simulink model "EVX_Lap_Simulation 2"  (R2018b)
settings: Solver=FixedStepAuto  StartTime=0  StopTime=120  FixedStep=0.001  MaxStep=0.01  RelTol=1e-2
values from neighbouring files (symbols this model uses):
  velocity_dnew = velocity_d + 0.4 .* (velocity_dmax - velocity_d)    [Run_Sim(with_fmincon).m]
undefined symbols (not defined in the file or in its folder): dist, theta_d
libraries: simulink x1
(part 2 of 3)

== system EVX_Lap_Simulation 2/EVX_Vehicle_Model/Subsystem1 ==
  Tyre Coefficients : Inport
  Tyre Dynamics : Inport  Port=2
  Bus Creator : BusCreator  Inputs=3
  Bus Selector : BusSelector  OutputSignals=Fzo,Ro,q_Bz1,q_Bz2,q_Bz3,q_Bz4,q_Bz5,q_Bz9,q_Bz10,q_Cz1,q_Dz1,q_Dz2,q_Dz3,q_Dz4,q_Dz6,q_Dz7,q_Dz8,q_Dz9,q_Ez1,q_Ez2,q_Ez3,q_Ez4,q_Ez5,q_Hz1,q_Hz2,q_Hz3,q_Hz4,p_Cy1,p_Dy1,p_Dy2,p_Dy3,p_Ey1,p_Ey2,p_Ey3,p_Ey4,p_Ky1,p_Ky2,p_Ky3,p_Hy1,p_Hy2,p_Hy3,p_Vy1,p_Vy2,p_Vy3,p_Vy4,p_Cx1,p_Dx1,p_Dx2,p_Ex1,p_Ex2,p_Ex3,p_Ex4,p_Kx1,p_Kx2,p_Kx3,p_Hx1,p_Hx2,p_Vx1,p_Vx2
  Bus Selector1 : BusSelector  OutputSignals=x_WFR,xdot_WFR,signal3.k_TFR,signal3.c_TFR,signal3.gamma_FR,signal4.ratio_FR,signal4.angle_FR,mu_scaling
  Constant : Constant  Value=0
  MATLAB Function : MATLAB Function  TreatAsAtomicUnit=on
  MATLAB Function8 : MATLAB Function  TreatAsAtomicUnit=on
  Memory1 : Memory
  Multiply : Product  Inputs=3
  Multiply1 : Product  Inputs=3
  Scope : Scope
  Scope1 : Scope  NumInputPorts=3
  Output Forces : Outport
  wires:
  Bus Creator/1 -> Scope/1, Output Forces/1
  Tyre Coefficients/1 -> Bus Selector/1
  Bus Selector/1 -> MATLAB Function8/5(Fzo)  "<Fzo>"
  Bus Selector/2 -> MATLAB Function8/6(Ro)  "<Ro>"
  Tyre Dynamics/1 -> Memory1/1
  Bus Selector1/1 -> MATLAB Function/1(x)  "<x_WFR>"
  Bus Selector1/2 -> MATLAB Function/2(xdot)  "<xdot_WFR>"
  MATLAB Function/1(F_z) -> Multiply1/2, Multiply/2, Scope1/1, MATLAB Function8/1(Fz)
  Bus Selector1/3 -> MATLAB Function/3(k)  "<k_TFR>"
  Bus Selector1/4 -> MATLAB Function/4(c)  "<c_TFR>"
  Bus Selector1/5 -> MATLAB Function8/4(gam)  "<gamma_FR>"
  Bus Selector/3 -> MATLAB Function8/7(q_Bz1)  "<q_Bz1>"
  Bus Selector/4 -> MATLAB Function8/8(q_Bz2)  "<q_Bz2>"
  Bus Selector/5 -> MATLAB Function8/9(q_Bz3)  "<q_Bz3>"
  Bus Selector/6 -> MATLAB Function8/10(q_Bz4)  "<q_Bz4>"
  Bus Selector/7 -> MATLAB Function8/11(q_Bz5)  "<q_Bz5>"
  Bus Selector/8 -> MATLAB Function8/12(q_Bz9)  "<q_Bz9>"
  Bus Selector/9 -> MATLAB Function8/13(q_Bz10)  "<q_Bz10>"
  Bus Selector/10 -> MATLAB Function8/14(q_Cz1)  "<q_Cz1>"
  Bus Selector/11 -> MATLAB Function8/15(q_Dz1)  "<q_Dz1>"
  Bus Selector/12 -> MATLAB Function8/16(q_Dz2)  "<q_Dz2>"
  Bus Selector/13 -> MATLAB Function8/17(q_Dz3)  "<q_Dz3>"
  Bus Selector/14 -> MATLAB Function8/18(q_Dz4)  "<q_Dz4>"
  Bus Selector/15 -> MATLAB Function8/19(q_Dz6)  "<q_Dz6>"
  Bus Selector/16 -> MATLAB Function8/20(q_Dz7)  "<q_Dz7>"
  Bus Selector/17 -> MATLAB Function8/21(q_Dz8)  "<q_Dz8>"
  Bus Selector/18 -> MATLAB Function8/22(q_Dz9)  "<q_Dz9>"
  Bus Selector/19 -> MATLAB Function8/23(q_Ez1)  "<q_Ez1>"
  Bus Selector/20 -> MATLAB Function8/24(q_Ez2)  "<q_Ez2>"
  Bus Selector/21 -> MATLAB Function8/25(q_Ez3)  "<q_Ez3>"
  Bus Selector/22 -> MATLAB Function8/26(q_Ez4)  "<q_Ez4>"
  Bus Selector/23 -> MATLAB Function8/27(q_Ez5)  "<q_Ez5>"
  Bus Selector/24 -> MATLAB Function8/28(q_Hz1)  "<q_Hz1>"
  Bus Selector/25 -> MATLAB Function8/29(q_Hz2)  "<q_Hz2>"
  Bus Selector/26 -> MATLAB Function8/30(q_Hz3)  "<q_Hz3>"
  Bus Selector/27 -> MATLAB Function8/31(q_Hz4)  "<q_Hz4>"
  Bus Selector/28 -> MATLAB Function8/32(p_Cy1)  "<p_Cy1>"
  Bus Selector/29 -> MATLAB Function8/33(p_Dy1)  "<p_Dy1>"
  Bus Selector/30 -> MATLAB Function8/34(p_Dy2)  "<p_Dy2>"
  Bus Selector/31 -> MATLAB Function8/35(p_Dy3)  "<p_Dy3>"
  Bus Selector/32 -> MATLAB Function8/36(p_Ey1)  "<p_Ey1>"
  Bus Selector/33 -> MATLAB Function8/37(p_Ey2)  "<p_Ey2>"
  Bus Selector/34 -> MATLAB Function8/38(p_Ey3)  "<p_Ey3>"
  Bus Selector/35 -> MATLAB Function8/39(p_Ey4)  "<p_Ey4>"
  Bus Selector/36 -> MATLAB Function8/40(p_Ky1)  "<p_Ky1>"
  Bus Selector/37 -> MATLAB Function8/41(p_Ky2)  "<p_Ky2>"
  Bus Selector/38 -> MATLAB Function8/42(p_Ky3)  "<p_Ky3>"
  Bus Selector/39 -> MATLAB Function8/43(p_Hy1)  "<p_Hy1>"
  Bus Selector/40 -> MATLAB Function8/44(p_Hy2)  "<p_Hy2>"
  Bus Selector/41 -> MATLAB Function8/45(p_Hy3)  "<p_Hy3>"
  Bus Selector/42 -> MATLAB Function8/46(p_Vy1)  "<p_Vy1>"
  Bus Selector/43 -> MATLAB Function8/47(p_Vy2)  "<p_Vy2>"
  Bus Selector/44 -> MATLAB Function8/48(p_Vy3)  "<p_Vy3>"
  Bus Selector/45 -> MATLAB Function8/49(p_Vy4)  "<p_Vy4>"
  Bus Selector/46 -> MATLAB Function8/50(p_Cx1)  "<p_Cx1>"
  Bus Selector/47 -> MATLAB Function8/51(p_Dx1)  "<p_Dx1>"
  Bus Selector/48 -> MATLAB Function8/52(p_Dx2)  "<p_Dx2>"
  Bus Selector/49 -> MATLAB Function8/53(p_Ex1)  "<p_Ex1>"
  Bus Selector/50 -> MATLAB Function8/54(p_Ex2)  "<p_Ex2>"
  Bus Selector/51 -> MATLAB Function8/55(p_Ex3)  "<p_Ex3>"
  Bus Selector/52 -> MATLAB Function8/56(p_Ex4)  "<p_Ex4>"
  Bus Selector/53 -> MATLAB Function8/57(p_Kx1)  "<p_Kx1>"
  Bus Selector/54 -> MATLAB Function8/58(p_Kx2)  "<p_Kx2>"
  Bus Selector/55 -> MATLAB Function8/59(p_Kx3)  "<p_Kx3>"
  Bus Selector/56 -> MATLAB Function8/60(p_Hx1)  "<p_Hx1>"
  Bus Selector/57 -> MATLAB Function8/61(p_Hx2)  "<p_Hx2>"
  Bus Selector/58 -> MATLAB Function8/62(p_Vx1)  "<p_Vx1>"
  Bus Selector/59 -> MATLAB Function8/63(p_Vx2)  "<p_Vx2>"
  Bus Selector1/8 -> Multiply1/1, Multiply/1, MATLAB Function8/64(car_mu_scaling)  "<mu_scaling>"
  Bus Selector1/6 -> Multiply/3, Scope1/2, MATLAB Function8/2(kappa)  "<ratio_FR>"
  Bus Selector1/7 -> Scope1/3, MATLAB Function8/3(alpha), Multiply1/3  "<angle_FR>"
  Memory1/1 -> Bus Selector1/1
  Multiply/1 -> Bus Creator/1  "Fxo"
  Multiply1/1 -> Bus Creator/2  "Fyo"
  Constant/1 -> Bus Creator/3  "Mzo"

== system EVX_Lap_Simulation 2/EVX_Vehicle_Model/Subsystem3 ==
  Steering Angle : Inport
  Bus Creator : BusCreator  Inputs=4
  Constant : Constant  Value=2
  Constant1 : Constant  Value=6
  Front/Rear Split : MATLAB Function  TreatAsAtomicUnit=on
  MATLAB Function : MATLAB Function  TreatAsAtomicUnit=on
  MATLAB Function1 : MATLAB Function  TreatAsAtomicUnit=on
  Wheel Angles : Outport
  wires:
  Steering Angle/1 -> Front/Rear Split/1(Angle)
  Front/Rear Split/1(Steering_F) -> MATLAB Function/1(Steering_F)
  Front/Rear Split/2(Steering_R) -> MATLAB Function1/1(Steering_R)
  Constant/1 -> MATLAB Function/2(Ratio)
  Constant1/1 -> MATLAB Function1/2(Ratio)
  MATLAB Function/1(S_FR) -> Bus Creator/1
  MATLAB Function1/1(S_RR) -> Bus Creator/3
  MATLAB Function1/2(S_RL) -> Bus Creator/4
  Bus Creator/1 -> Wheel Angles/1
  MATLAB Function/2(S_FL) -> Bus Creator/2

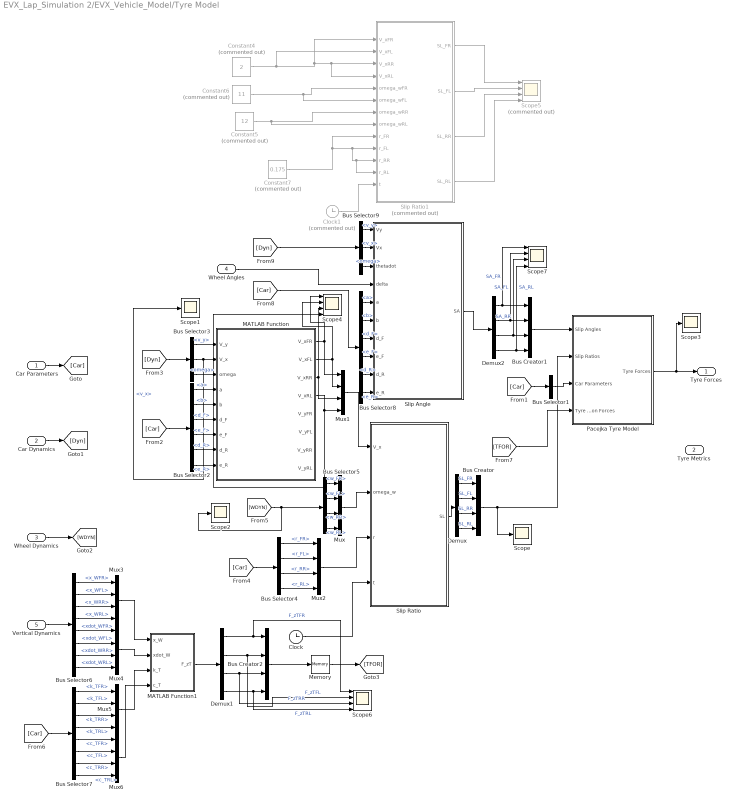
== system EVX_Lap_Simulation 2/EVX_Vehicle_Model/Tyre Model ==
  Car Parameters : Inport
  Car Dynamics : Inport  Port=2
  Wheel Dynamics : Inport  Port=3
  Wheel Angles : Inport  Port=4
  Vertical Dynamics : Inport  Port=5
  Bus Creator : BusCreator  Inputs=4
  Bus Creator1 : BusCreator  Inputs=4
  Bus Creator2 : BusCreator  Inputs=4
  Bus Selector1 : BusSelector  OutputSignals=Chassis Param,Suspension Param  OutputAsBus=on
  Bus Selector2 : BusSelector  OutputSignals=Chassis Param.a,Chassis Param.b,Chassis Param.d_F,Chassis Param.e_F,Chassis Param.d_R,Chassis Param.e_R
  Bus Selector3 : BusSelector  OutputSignals=Car Velocities.v_y,Car Velocities.v_x,Car Velocities.omega
  Bus Selector4 : BusSelector  OutputSignals=Wheel Param.r_FR,Wheel Param.r_FL,Wheel Param.r_RR,Wheel Param.r_RL
  Bus Selector5 : BusSelector  OutputSignals=w.w_FR,w.w_FL,w.w_RR,w.w_RL
  Bus Selector6 : BusSelector  OutputSignals=V_Disp.x_WFR,V_Disp.x_WFL,V_Disp.x_WRR,V_Disp.x_WRL,V_Vel.xdot_WFR,V_Vel.xdot_WFL,V_Vel.xdot_WRR,V_Vel.xdot_WRL
  Bus Selector7 : BusSelector  OutputSignals=Suspension Param.k_TFR,Suspension Param.k_TFL,Suspension Param.k_TRR,Suspension Param.k_TRL,Suspension Param.c_TFR,Suspension Param.c_TFL,Suspension Param.c_TRR,Suspension Param.c_TRL
  Bus Selector8 : BusSelector  OutputSignals=Chassis Param.a,Chassis Param.b,Chassis Param.d_F,Chassis Param.e_F,Chassis Param.d_R,Chassis Param.e_R
  Bus Selector9 : BusSelector  OutputSignals=Car Velocities.v_y,Car Velocities.v_x,Car Velocities.omega
  Clock : Clock
  Clock1 : Clock  Commented=on
  Constant4 : Constant  Commented=on  Value=2
  Constant5 : Constant  Commented=on  Value=12
  Constant6 : Constant  Commented=on  Value=11
  Constant7 : Constant  Commented=on  Value=0.175
  Demux : Demux
  Demux1 : Demux
  Demux2 : Demux
  MATLAB Function : MATLAB Function  TreatAsAtomicUnit=on
  MATLAB Function1 : MATLAB Function  TreatAsAtomicUnit=on
  Memory : Memory
  Mux{,1..6} (7 alike) : Mux
  Pacejka Tyre Model : Subsystem
  Scope{,1..3} (4 alike) : Scope
  Scope4 : Scope  NumInputPorts=4
  Scope5 : Scope  Commented=on  NumInputPorts=4
  Scope6 : Scope  NumInputPorts=4
  Scope7 : Scope  NumInputPorts=4
  Slip Angle : MATLAB Function  TreatAsAtomicUnit=on
  Slip Ratio : MATLAB Function  TreatAsAtomicUnit=on
  Slip Ratio1 : MATLAB Function  Commented=on  TreatAsAtomicUnit=on
  Tyre Forces : Outport
  Tyre Metrics : Outport  Port=2
  wires:
  Car Parameters/1 -> [Car]
  [Car] -> Bus Selector1/1
  [Car] -> Bus Selector2/1
  Bus Selector2/1 -> MATLAB Function/4(a)  "<a>"
  Bus Selector2/2 -> MATLAB Function/5(b)  "<b>"
  Bus Selector2/3 -> MATLAB Function/6(d_F)  "<d_F>"
  Bus Selector2/4 -> MATLAB Function/7(e_F)  "<e_F>"
  Bus Selector2/5 -> MATLAB Function/8(d_R)  "<d_R>"
  Bus Selector2/6 -> MATLAB Function/9(e_R)  "<e_R>"
  Car Dynamics/1 -> [Dyn]
  [Dyn] -> Bus Selector3/1
  Bus Selector3/3 -> MATLAB Function/3(omega)  "<omega>"
  Bus Selector3/1 -> MATLAB Function/1(V_y)  "<v_y>"
  Bus Selector3/2 -> Scope1/1, MATLAB Function/2(V_x)  "<v_x>"
  MATLAB Function/1(V_xFR) -> Scope4/1, Mux1/1
  MATLAB Function/2(V_xFL) -> Scope4/2, Mux1/2
  MATLAB Function/3(V_xRR) -> Scope4/3, Mux1/3
  MATLAB Function/4(V_xRL) -> Mux1/4, Scope4/4
  [Car] -> Bus Selector4/1
  Wheel Dynamics/1 -> [WDYN]
  [WDYN] -> Scope2/1, Bus Selector5/1
  Pacejka Tyre Model/1(Tyre Forces) -> Scope3/1, Tyre Forces/1
  Bus Selector1/1 -> Pacejka Tyre Model/3(Car Parameters)
  Bus Creator/1 -> Scope/1, Pacejka Tyre Model/2(Slip Ratios)
  Bus Creator1/1 -> Pacejka Tyre Model/1(Slip Angles)
  [TFOR] -> Pacejka Tyre Model/4(Tyre Reaction Forces)
  Clock/1 -> Slip Ratio/4(t)
  Constant4/1 -> Slip Ratio1/2(V_xFL), Slip Ratio1/1(V_xFR), Slip Ratio1/4(V_xRL), Slip Ratio1/3(V_xRR)
  Constant5/1 -> Slip Ratio1/8(omega_wRL), Slip Ratio1/7(omega_wRR)
  Constant6/1 -> Slip Ratio1/6(omega_wFL), Slip Ratio1/5(omega_wFR)
  Constant7/1 -> Slip Ratio1/12(r_RL), Slip Ratio1/11(r_RR), Slip Ratio1/10(r_FL), Slip Ratio1/9(r_FR)
  Clock1/1 -> Slip Ratio1/13(t)
  Slip Ratio1/1(SL_FR) -> Scope5/1
  Slip Ratio1/2(SL_FL) -> Scope5/2
  Slip Ratio1/3(SL_RR) -> Scope5/3
  Slip Ratio1/4(SL_RL) -> Scope5/4
  Bus Selector5/4 -> Mux/4  "<w_RL>"
  Bus Selector5/1 -> Mux/1  "<w_FR>"
  Bus Selector5/2 -> Mux/2  "<w_FL>"
  Bus Selector5/3 -> Mux/3  "<w_RR>"
  Mux/1 -> Slip Ratio/2(omega_w)
  Mux1/1 -> Slip Ratio/1(V_x)
  Bus Selector4/1 -> Mux2/1  "<r_FR>"
  Bus Selector4/2 -> Mux2/2  "<r_FL>"
  Bus Selector4/3 -> Mux2/3  "<r_RR>"
  Bus Selector4/4 -> Mux2/4  "<r_RL>"
  Mux2/1 -> Slip Ratio/3(r)
  Slip Ratio/1(SL) -> Demux/1
  Demux/1 -> Bus Creator/1  "SL_FR"
  Demux/2 -> Bus Creator/2  "SL_FL"
  Demux/3 -> Bus Creator/3  "SL_RR"
  Demux/4 -> Bus Creator/4  "SL_RL"
  Vertical Dynamics/1 -> Bus Selector6/1
  Bus Selector6/1 -> Mux3/1  "<x_WFR>"
  Bus Selector6/2 -> Mux3/2  "<x_WFL>"
  Bus Selector6/3 -> Mux3/3  "<x_WRR>"
  Bus Selector6/4 -> Mux3/4  "<x_WRL>"
  Bus Selector6/5 -> Mux4/1  "<xdot_WFR>"
  Bus Selector6/6 -> Mux4/2  "<xdot_WFL>"
  Bus Selector6/7 -> Mux4/3  "<xdot_WRR>"
  Bus Selector6/8 -> Mux4/4  "<xdot_WRL>"
  [Car] -> Bus Selector7/1
  Bus Selector7/1 -> Mux5/1  "<k_TFR>"
  Bus Selector7/2 -> Mux5/2  "<k_TFL>"
  Bus Selector7/3 -> Mux5/3  "<k_TRR>"
  Bus Selector7/4 -> Mux5/4  "<k_TRL>"
  Bus Selector7/5 -> Mux6/1  "<c_TFR>"
  Bus Selector7/6 -> Mux6/2  "<c_TFL>"
  Bus Selector7/7 -> Mux6/3  "<c_TRR>"
  Bus Selector7/8 -> Mux6/4  "<c_TRL>"
  Mux3/1 -> MATLAB Function1/1(x_W)
  Mux4/1 -> MATLAB Function1/2(xdot_W)
  Mux5/1 -> MATLAB Function1/3(k_T)
  Mux6/1 -> MATLAB Function1/4(c_T)
  MATLAB Function1/1(F_zT) -> Demux1/1
  Demux1/1 -> Scope6/1, Bus Creator2/1  "F_zTFR"
  Demux1/2 -> Scope6/2, Bus Creator2/2  "F_zTFL"
  Demux1/3 -> Scope6/3, Bus Creator2/3  "F_zTRR"
  Demux1/4 -> Scope6/4, Bus Creator2/4  "F_zTRL"
  Bus Creator2/1 -> Memory/1
  Memory/1 -> [TFOR]
  [Car] -> Bus Selector8/1
  Bus Selector8/1 -> Slip Angle/5(a)  "<a>"
  Bus Selector8/2 -> Slip Angle/6(b)  "<b>"
  Bus Selector8/3 -> Slip Angle/7(d_F)  "<d_F>"
  Bus Selector8/4 -> Slip Angle/8(e_F)  "<e_F>"
  Bus Selector8/5 -> Slip Angle/9(d_R)  "<d_R>"
  Bus Selector8/6 -> Slip Angle/10(e_R)  "<e_R>"
  [Dyn] -> Bus Selector9/1
  Bus Selector9/3 -> Slip Angle/3(thetadot)  "<omega>"
  Wheel Angles/1 -> Slip Angle/4(delta)
  Slip Angle/1(SA) -> Demux2/1
  Demux2/1 -> Scope7/1, Bus Creator1/1  "SA_FR"
  Demux2/2 -> Scope7/2, Bus Creator1/2  "SA_FL"
  Demux2/3 -> Scope7/3, Bus Creator1/3  "SA_RR"
  Demux2/4 -> Scope7/4, Bus Creator1/4  "SA_RL"
  Bus Selector9/2 -> Slip Angle/2(Vx)  "<v_x>"
  Bus Selector9/1 -> Slip Angle/1(Vy)  "<v_y>"

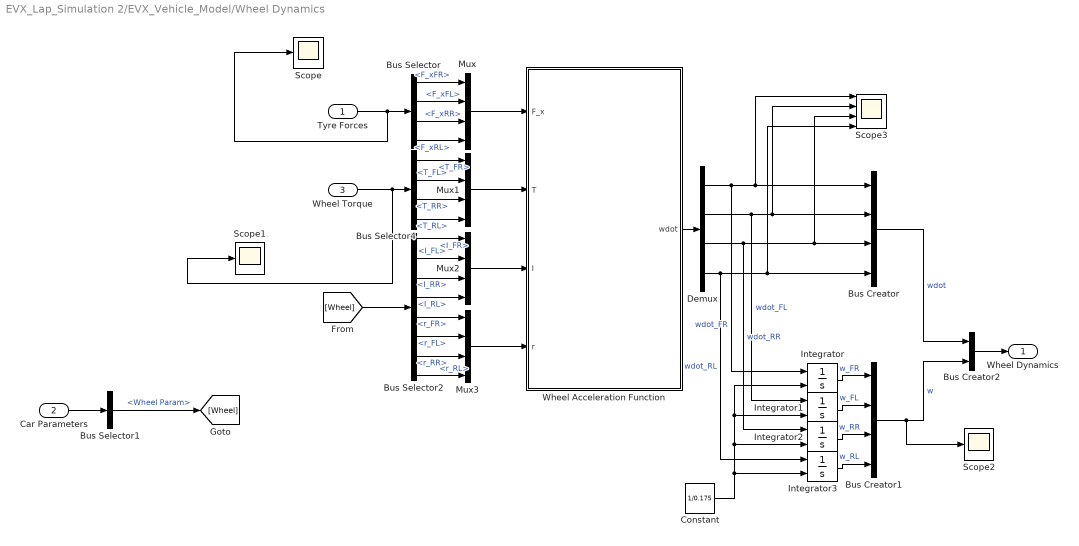
== system EVX_Lap_Simulation 2/EVX_Vehicle_Model/Wheel Dynamics ==
  Tyre Forces : Inport
  Car Parameters : Inport  Port=2
  Wheel Torque : Inport  Port=3
  Bus Creator : BusCreator  Inputs=4
  Bus Creator1 : BusCreator  Inputs=4
  Bus Creator2 : BusCreator  Inputs=2
  Bus Selector : BusSelector  OutputSignals=F_x.F_xFR,F_x.F_xFL,F_x.F_xRR,F_x.F_xRL
  Bus Selector1 : BusSelector  OutputSignals=Wheel Param
  Bus Selector2 : BusSelector  OutputSignals=I_FR,I_FL,I_RR,I_RL,r_FR,r_FL,r_RR,r_RL
  Bus Selector4 : BusSelector  OutputSignals=T_FR,T_FL,T_RR,T_RL
  Constant : Constant  Value=1/0.175
  Demux : Demux
  Integrator{,1..3} (4 alike) : Integrator  InitialConditionSource=external
  Mux{,1..3} (4 alike) : Mux
  Scope : Scope
  Scope1 : Scope
  Scope2 : Scope
  Scope3 : Scope  NumInputPorts=4
  Wheel Acceleration Function : MATLAB Function  TreatAsAtomicUnit=on
  Wheel Dynamics : Outport
  wires:
  Tyre Forces/1 -> Scope/1, Bus Selector/1
  Car Parameters/1 -> Bus Selector1/1
  Bus Selector1/1 -> [Wheel]  "<Wheel Param>"
  [Wheel] -> Bus Selector2/1
  Wheel Torque/1 -> Scope1/1, Bus Selector4/1
  Integrator/1 -> Bus Creator1/1  "w_FR"
  Integrator1/1 -> Bus Creator1/2  "w_FL"
  Integrator2/1 -> Bus Creator1/3  "w_RR"
  Integrator3/1 -> Bus Creator1/4  "w_RL"
  Bus Creator1/1 -> Scope2/1, Bus Creator2/2  "w"
  Bus Creator/1 -> Bus Creator2/1  "wdot"
  Bus Creator2/1 -> Wheel Dynamics/1
  Constant/1 -> Integrator3/2, Integrator2/2, Integrator1/2, Integrator/2
  Bus Selector/1 -> Mux/1  "<F_xFR>"
  Bus Selector/2 -> Mux/2  "<F_xFL>"
  Bus Selector/3 -> Mux/3  "<F_xRR>"
  Bus Selector/4 -> Mux/4  "<F_xRL>"
  Mux/1 -> Wheel Acceleration Function/1(F_x)
  Bus Selector4/2 -> Mux1/2  "<T_FL>"
  Bus Selector4/3 -> Mux1/3  "<T_RR>"
  Bus Selector4/4 -> Mux1/4  "<T_RL>"
  Bus Selector4/1 -> Mux1/1  "<T_FR>"
  Mux1/1 -> Wheel Acceleration Function/2(T)
  Bus Selector2/2 -> Mux2/2  "<I_FL>"
  Bus Selector2/3 -> Mux2/3  "<I_RR>"
  Bus Selector2/4 -> Mux2/4  "<I_RL>"
  Bus Selector2/1 -> Mux2/1  "<I_FR>"
  Mux2/1 -> Wheel Acceleration Function/3(I)
  Bus Selector2/5 -> Mux3/1  "<r_FR>"
  Bus Selector2/6 -> Mux3/2  "<r_FL>"
  Bus Selector2/7 -> Mux3/3  "<r_RR>"
  Bus Selector2/8 -> Mux3/4  "<r_RL>"
  Mux3/1 -> Wheel Acceleration Function/4(r)
  Wheel Acceleration Function/1(wdot) -> Demux/1
  Demux/1 -> Integrator/1, Scope3/1, Bus Creator/1  "wdot_FR"
  Demux/2 -> Integrator1/1, Scope3/2, Bus Creator/2  "wdot_FL"
  Demux/3 -> Integrator2/1, Scope3/3, Bus Creator/3  "wdot_RR"
  Demux/4 -> Integrator3/1, Scope3/4, Bus Creator/4  "wdot_RL"

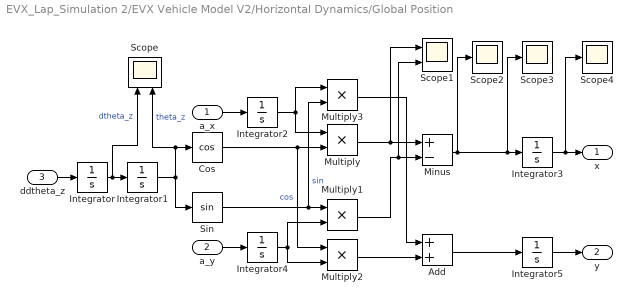
== system EVX_Lap_Simulation 2/EVX Vehicle Model V2/Horizontal Dynamics/Global Position ==
  a_x : Inport
  a_y : Inport  Port=2
  ddtheta_z : Inport  Port=3
  Add : Sum
  Cos : Trigonometry  Operator=cos
  Integrator{,1..5} (6 alike) : Integrator
  Minus : Sum  Inputs=+-
  Multiply{,1..3} (4 alike) : Product
  Scope : Scope  NumInputPorts=2
  Scope1 : Scope  NumInputPorts=2
  Scope2 : Scope
  Scope3 : Scope
  Scope4 : Scope
  Sin : Trigonometry
  x : Outport
  y : Outport  Port=2
  wires:
  ddtheta_z/1 -> Integrator/1
  Integrator/1 -> Scope/1, Integrator1/1  "dtheta_z"
  Integrator1/1 -> Scope/2, Cos/1, Sin/1  "theta_z"
  a_x/1 -> Integrator2/1
  Cos/1 -> Multiply2/1, Multiply/2  "cos"
  Sin/1 -> Multiply3/2, Multiply1/1  "sin"
  a_y/1 -> Integrator4/1
  Multiply/1 -> Scope1/1, Minus/1
  Multiply1/1 -> Scope1/2, Minus/2
  Multiply2/1 -> Add/2
  Multiply3/1 -> Add/1
  Minus/1 -> Scope3/1, Integrator3/1, Scope2/1
  Integrator3/1 -> Scope4/1, x/1
  Add/1 -> Integrator5/1
  Integrator5/1 -> y/1
  Integrator2/1 -> Multiply/1, Multiply3/1
  Integrator4/1 -> Multiply2/2, Multiply1/2

== system EVX_Lap_Simulation 2/EVX Vehicle Model V2/Horizontal Dynamics/Local Dynamics ==
  a_x : Inport
  a_y : Inport  Port=2
  ddtheta_z : Inport  Port=3
  Bus Creator{,1..3} (4 alike) : BusCreator  Inputs=3
  Integrator{,1..5} (6 alike) : Integrator
  Scope{,1..3} (4 alike) : Scope
  To Workspace : ToWorkspace  VariableName=dist_log  SaveFormat=Timeseries  SampleTime=-1
  Local Dynamics : Outport
  wires:
  Integrator/1 -> Bus Creator1/1, Scope/1, Integrator3/1  "v_x"
  Integrator2/1 -> Scope3/1, Bus Creator1/3, Integrator5/1  "dtheta_z"
  Integrator1/1 -> Bus Creator1/2, Scope2/1, Integrator4/1  "v_y"
  a_x/1 -> Bus Creator/1, Integrator/1
  a_y/1 -> Bus Creator/2, Integrator1/1
  ddtheta_z/1 -> Bus Creator/3, Integrator2/1
  Integrator4/1 -> Bus Creator2/2  "d_y"
  Integrator3/1 -> To Workspace/1, Scope1/1, Bus Creator2/1  "d_x"
  Integrator5/1 -> Bus Creator2/3  "theta_z"
  Bus Creator1/1 -> Bus Creator3/2  "Velocities"
  Bus Creator/1 -> Bus Creator3/1  "Accelerations"
  Bus Creator2/1 -> Bus Creator3/3  "Displacements"
  Bus Creator3/1 -> Local Dynamics/1

== system EVX_Lap_Simulation 2/EVX Vehicle Model V2/Tyre Model/Pacejka Tyre Model ==
  Slip Ratios : Inport
  Slip Angles : Inport  Port=2
  Tyre Reaction Forces : Inport  Port=3
  Bus Creator : BusCreator  Inputs=3
  Demux : Demux
  Demux1 : Demux
  Demux2 : Demux
  MATLAB Function4 : MATLAB Function  TreatAsAtomicUnit=on
  Scope : Scope  NumInputPorts=4
  Scope1 : Scope
  Scope2 : Scope  NumInputPorts=4
  Scope3 : Scope  NumInputPorts=4
  To Workspace : ToWorkspace  VariableName=Fz_log  SaveFormat=Timeseries  SampleTime=-1
  Tyre Forces : Outport
  wires:
  Bus Creator/1 -> Tyre Forces/1
  Slip Ratios/1 -> MATLAB Function4/2(SL)
  Slip Angles/1 -> MATLAB Function4/1(SA)
  Tyre Reaction Forces/1 -> To Workspace/1, Scope1/1, MATLAB Function4/3(Fz)
  MATLAB Function4/1(F_x) -> Demux/1, Bus Creator/1
  MATLAB Function4/2(F_y) -> Demux2/1, Bus Creator/2
  MATLAB Function4/3(M_z) -> Demux1/1, Bus Creator/3
  Demux/1 -> Scope/1  "F_xFL"
  Demux/2 -> Scope/2  "F_xFR"
  Demux/3 -> Scope/3  "F_xRL"
  Demux/4 -> Scope/4  "F_xRR"
  Demux1/1 -> Scope2/1  "M_zFL"
  Demux1/2 -> Scope2/2  "M_zFR"
  Demux1/3 -> Scope2/3  "M_zRL"
  Demux1/4 -> Scope2/4  "M_zRR"
  Demux2/1 -> Scope3/1  "F_yFL"
  Demux2/2 -> Scope3/2  "F_yFR"
  Demux2/3 -> Scope3/3  "F_yRL"
  Demux2/4 -> Scope3/4  "F_yRR"

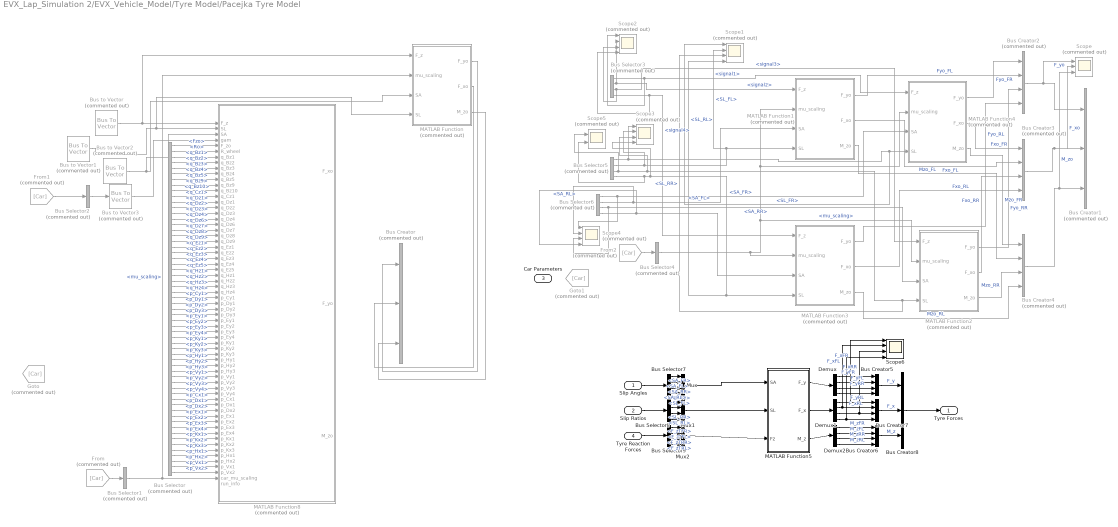
== system EVX_Lap_Simulation 2/EVX_Vehicle_Model/Tyre Model/Pacejka Tyre Model ==
  Slip Angles : Inport
  Slip Ratios : Inport  Port=2
  Car Parameters : Inport  Port=3
  Tyre Reaction Forces : Inport  Port=4
  Bus Creator : BusCreator  Commented=on  Inputs=3
  Bus Creator1 : BusCreator  Commented=on  Inputs=3
  Bus Creator2 : BusCreator  Commented=on  Inputs=4
  Bus Creator3 : BusCreator  Commented=on  Inputs=4
  Bus Creator4 : BusCreator  Commented=on  Inputs=4
  Bus Creator5 : BusCreator  Inputs=4
  Bus Creator6 : BusCreator  Inputs=4
  Bus Creator7 : BusCreator  Inputs=4
  Bus Creator8 : BusCreator  Inputs=3
  Bus Selector : BusSelector  Commented=on  OutputSignals=Fzo,Ro,q_Bz1,q_Bz2,q_Bz3,q_Bz4,q_Bz5,q_Bz9,q_Bz10,q_Cz1,q_Dz1,q_Dz2,q_Dz3,q_Dz4,q_Dz6,q_Dz7,q_Dz8,q_Dz9,q_Ez1,q_Ez2,q_Ez3,q_Ez4,q_Ez5,q_Hz1,q_Hz2,q_Hz3,q_Hz4,p_Cy1,p_Dy1,p_Dy2,p_Dy3,p_Ey1,p_Ey2,p_Ey3,p_Ey4,p_Ky1,p_Ky2,p_Ky3,p_Hy1,p_Hy2,p_Hy3,p_Vy1,p_Vy2,p_Vy3,p_Vy4,p_Cx1,p_Dx1,p_Dx2,p_Ex1,p_Ex2,p_Ex3,p_Ex4,p_Kx1,p_Kx2,p_Kx3,p_Hx1,p_Hx2,p_Vx1,p_Vx2
  Bus Selector1 : BusSelector  Commented=on  OutputSignals=Chassis Param.mu_scaling
  Bus Selector2 : BusSelector  Commented=on  OutputSignals=Suspension Param.gamma_FR,Suspension Param.gamma_FL,Suspension Param.gamma_RR,Suspension Param.gamma_RL  OutputAsBus=on
  Bus Selector3 : BusSelector  Commented=on  OutputSignals=signal1,signal2,signal3,signal4
  Bus Selector4 : BusSelector  Commented=on  OutputSignals=Chassis Param.mu_scaling
  Bus Selector5 : BusSelector  Commented=on  OutputSignals=SL_FR,SL_FL,SL_RR,SL_RL
  Bus Selector6 : BusSelector  Commented=on  OutputSignals=SA_FR,SA_FL,SA_RR,SA_RL
  Bus Selector7 : BusSelector  OutputSignals=SA_FR,SA_FL,SA_RR,SA_RL
  Bus Selector8 : BusSelector  OutputSignals=SL_FR,SL_FL,SL_RR,SL_RL
  Bus Selector9 : BusSelector  OutputSignals=F_zTFR,F_zTFL,F_zTRR,F_zTRL
  Bus to Vector{,1..3} (4 alike) : BusToVector  Commented=on
  Demux : Demux
  Demux1 : Demux
  Demux2 : Demux
  From : From  Commented=on  GotoTag=Car
  From1 : From  Commented=on  GotoTag=Car
  From2 : From  Commented=on  GotoTag=Car
  Goto : Goto  Commented=on  GotoTag=Car
  Goto1 : Goto  Commented=on  GotoTag=Car
  MATLAB Function : MATLAB Function  Commented=on  TreatAsAtomicUnit=on
  MATLAB Function1 : MATLAB Function  Commented=on  TreatAsAtomicUnit=on
  MATLAB Function2 : MATLAB Function  Commented=on  TreatAsAtomicUnit=on
  MATLAB Function3 : MATLAB Function  Commented=on  TreatAsAtomicUnit=on
  MATLAB Function4 : MATLAB Function  Commented=on  TreatAsAtomicUnit=on
  MATLAB Function5 : MATLAB Function  TreatAsAtomicUnit=on
  MATLAB Function8 : MATLAB Function  Commented=on  TreatAsAtomicUnit=on
  Mux : Mux
  Mux1 : Mux
  Mux2 : Mux
  Scope : Scope  Commented=on  NumInputPorts=3
  Scope{1..4} (4 alike) : Scope  Commented=on  NumInputPorts=4
  Scope5 : Scope  Commented=on  NumInputPorts=2
  Scope6 : Scope  NumInputPorts=4
  Tyre Forces : Outport
  wires:
  Bus Selector/1 -> MATLAB Function8/5(F_zo)  "<Fzo>"
  Bus Selector/2 -> MATLAB Function8/6(R_wheel)  "<Ro>"
  Bus Selector/3 -> MATLAB Function8/7(q_Bz1)  "<q_Bz1>"
  Bus Selector/4 -> MATLAB Function8/8(q_Bz2)  "<q_Bz2>"
  Bus Selector/5 -> MATLAB Function8/9(q_Bz3)  "<q_Bz3>"
  Bus Selector/6 -> MATLAB Function8/10(q_Bz4)  "<q_Bz4>"
  Bus Selector/7 -> MATLAB Function8/11(q_Bz5)  "<q_Bz5>"
  Bus Selector/8 -> MATLAB Function8/12(q_Bz9)  "<q_Bz9>"
  Bus Selector/9 -> MATLAB Function8/13(q_Bz10)  "<q_Bz10>"
  Bus Selector/10 -> MATLAB Function8/14(q_Cz1)  "<q_Cz1>"
  Bus Selector/11 -> MATLAB Function8/15(q_Dz1)  "<q_Dz1>"
  Bus Selector/12 -> MATLAB Function8/16(q_Dz2)  "<q_Dz2>"
  Bus Selector/13 -> MATLAB Function8/17(q_Dz3)  "<q_Dz3>"
  Bus Selector/14 -> MATLAB Function8/18(q_Dz4)  "<q_Dz4>"
  Bus Selector/15 -> MATLAB Function8/19(q_Dz6)  "<q_Dz6>"
  Bus Selector/16 -> MATLAB Function8/20(q_Dz7)  "<q_Dz7>"
  Bus Selector/17 -> MATLAB Function8/21(q_Dz8)  "<q_Dz8>"
  Bus Selector/18 -> MATLAB Function8/22(q_Dz9)  "<q_Dz9>"
  Bus Selector/19 -> MATLAB Function8/23(q_Ez1)  "<q_Ez1>"
  Bus Selector/20 -> MATLAB Function8/24(q_Ez2)  "<q_Ez2>"
  Bus Selector/21 -> MATLAB Function8/25(q_Ez3)  "<q_Ez3>"
  Bus Selector/22 -> MATLAB Function8/26(q_Ez4)  "<q_Ez4>"
  Bus Selector/23 -> MATLAB Function8/27(q_Ez5)  "<q_Ez5>"
  Bus Selector/24 -> MATLAB Function8/28(q_Hz1)  "<q_Hz1>"
  Bus Selector/25 -> MATLAB Function8/29(q_Hz2)  "<q_Hz2>"
  Bus Selector/26 -> MATLAB Function8/30(q_Hz3)  "<q_Hz3>"
  Bus Selector/27 -> MATLAB Function8/31(q_Hz4)  "<q_Hz4>"
  Bus Selector/28 -> MATLAB Function8/32(p_Cy1)  "<p_Cy1>"
  Bus Selector/29 -> MATLAB Function8/33(p_Dy1)  "<p_Dy1>"
  Bus Selector/30 -> MATLAB Function8/34(p_Dy2)  "<p_Dy2>"
  Bus Selector/31 -> MATLAB Function8/35(p_Dy3)  "<p_Dy3>"
  Bus Selector/32 -> MATLAB Function8/36(p_Ey1)  "<p_Ey1>"
  Bus Selector/33 -> MATLAB Function8/37(p_Ey2)  "<p_Ey2>"
  Bus Selector/34 -> MATLAB Function8/38(p_Ey3)  "<p_Ey3>"
  Bus Selector/35 -> MATLAB Function8/39(p_Ey4)  "<p_Ey4>"
  Bus Selector/36 -> MATLAB Function8/40(p_Ky1)  "<p_Ky1>"
  Bus Selector/37 -> MATLAB Function8/41(p_Ky2)  "<p_Ky2>"
  Bus Selector/38 -> MATLAB Function8/42(p_Ky3)  "<p_Ky3>"
  Bus Selector/39 -> MATLAB Function8/43(p_Hy1)  "<p_Hy1>"
  Bus Selector/40 -> MATLAB Function8/44(p_Hy2)  "<p_Hy2>"
  Bus Selector/41 -> MATLAB Function8/45(p_Hy3)  "<p_Hy3>"
  Bus Selector/42 -> MATLAB Function8/46(p_Vy1)  "<p_Vy1>"
  Bus Selector/43 -> MATLAB Function8/47(p_Vy2)  "<p_Vy2>"
  Bus Selector/44 -> MATLAB Function8/48(p_Vy3)  "<p_Vy3>"
  Bus Selector/45 -> MATLAB Function8/49(p_Vy4)  "<p_Vy4>"
  Bus Selector/46 -> MATLAB Function8/50(p_Cx1)  "<p_Cx1>"
  Bus Selector/47 -> MATLAB Function8/51(p_Dx1)  "<p_Dx1>"
  Bus Selector/48 -> MATLAB Function8/52(p_Dx2)  "<p_Dx2>"
  Bus Selector/49 -> MATLAB Function8/53(p_Ex1)  "<p_Ex1>"
  Bus Selector/50 -> MATLAB Function8/54(p_Ex2)  "<p_Ex2>"
  Bus Selector/51 -> MATLAB Function8/55(p_Ex3)  "<p_Ex3>"
  Bus Selector/52 -> MATLAB Function8/56(p_Ex4)  "<p_Ex4>"
  Bus Selector/53 -> MATLAB Function8/57(p_Kx1)  "<p_Kx1>"
  Bus Selector/54 -> MATLAB Function8/58(p_Kx2)  "<p_Kx2>"
  Bus Selector/55 -> MATLAB Function8/59(p_Kx3)  "<p_Kx3>"
  Bus Selector/56 -> MATLAB Function8/60(p_Hx1)  "<p_Hx1>"
  Bus Selector/57 -> MATLAB Function8/61(p_Hx2)  "<p_Hx2>"
  Bus Selector/58 -> MATLAB Function8/62(p_Vx1)  "<p_Vx1>"
  Bus Selector/59 -> MATLAB Function8/63(p_Vx2)  "<p_Vx2>"
  Bus Selector1/1 -> MATLAB Function/2(mu_scaling), MATLAB Function8/64(car_mu_scaling)  "<mu_scaling>"
  From/1 -> Bus Selector1/1
  From1/1 -> Bus Selector2/1
  Bus Selector2/1 -> Bus to Vector3/1
  Bus to Vector/1 -> MATLAB Function/1(F_z), MATLAB Function8/1(F_z)
  Bus to Vector1/1 -> MATLAB Function/4(SL), MATLAB Function8/2(SL)
  Bus to Vector2/1 -> MATLAB Function/3(SA), MATLAB Function8/3(SA)
  Bus to Vector3/1 -> MATLAB Function8/4(gam)
  MATLAB Function/1(F_yo) -> Bus Creator/1
  MATLAB Function/2(F_xo) -> Bus Creator/2
  MATLAB Function/3(M_zo) -> Bus Creator/3
  Bus Selector4/1 -> MATLAB Function3/2(mu_scaling), MATLAB Function2/2(mu_scaling), MATLAB Function1/2(mu_scaling), MATLAB Function4/2(mu_scaling)  "<mu_scaling>"
  From2/1 -> Bus Selector4/1
  Bus Selector5/1 -> Scope3/1, Scope1/1, MATLAB Function4/4(SL)  "<SL_FR>"
  Bus Selector5/2 -> Scope3/2, MATLAB Function1/4(SL), Scope1/2  "<SL_FL>"
  Bus Selector5/3 -> Scope1/3, MATLAB Function2/4(SL), Scope3/3, Scope5/1  "<SL_RR>"
  Bus Selector5/4 -> Scope5/2, Scope3/4, MATLAB Function3/4(SL), Scope1/4  "<SL_RL>"
  Bus Selector6/1 -> Scope4/1, MATLAB Function4/3(SA)  "<SA_FR>"
  Bus Selector6/2 -> Scope4/2, MATLAB Function1/3(SA)  "<SA_FL>"
  Bus Selector6/3 -> MATLAB Function2/3(SA), Scope4/3  "<SA_RR>"
  Bus Selector6/4 -> Scope4/4, MATLAB Function3/3(SA)  "<SA_RL>"
  MATLAB Function4/1(F_yo) -> Bus Creator2/1  "Fyo_FR"
  MATLAB Function1/1(F_yo) -> Bus Creator2/2  "Fyo_FL"
  MATLAB Function2/1(F_yo) -> Bus Creator2/3  "Fyo_RR"
  MATLAB Function3/1(F_yo) -> Bus Creator2/4  "Fyo_RL"
  MATLAB Function4/2(F_xo) -> Bus Creator3/1  "Fxo_FR"
  MATLAB Function1/2(F_xo) -> Bus Creator3/2  "Fxo_FL"
  MATLAB Function2/2(F_xo) -> Bus Creator3/3  "Fxo_RR"
  MATLAB Function3/2(F_xo) -> Bus Creator3/4  "Fxo_RL"
  MATLAB Function4/3(M_zo) -> Bus Creator4/1  "Mzo_FR"
  MATLAB Function1/3(M_zo) -> Bus Creator4/2  "Mzo_FL"
  MATLAB Function2/3(M_zo) -> Bus Creator4/3  "Mzo_RR"
  MATLAB Function3/3(M_zo) -> Bus Creator4/4  "Mzo_RL"
  Bus Creator3/1 -> Scope/2, Bus Creator1/2  "F_xo"
  Bus Creator2/1 -> Scope/1, Bus Creator1/1  "F_yo"
  Bus Creator4/1 -> Scope/3, Bus Creator1/3  "M_zo"
  Bus Selector3/1 -> Scope2/1, MATLAB Function4/1(F_z)  "<signal1>"
  Bus Selector3/2 -> Scope2/2, MATLAB Function1/1(F_z)  "<signal2>"
  Bus Selector3/3 -> Scope2/3, MATLAB Function2/1(F_z)  "<signal3>"
  Bus Selector3/4 -> Scope2/4, MATLAB Function3/1(F_z)  "<signal4>"
  Slip Angles/1 -> Bus Selector7/1
  Bus Selector8/2 -> Mux1/2  "<SL_FL>"
  Slip Ratios/1 -> Bus Selector8/1
  Bus Selector8/1 -> Mux1/1  "<SL_FR>"
  Bus Selector8/3 -> Mux1/3  "<SL_RR>"
  Bus Selector8/4 -> Mux1/4  "<SL_RL>"
  Bus Selector9/2 -> Mux2/2  "<F_zTFL>"
  Tyre Reaction Forces/1 -> Bus Selector9/1
  Bus Selector9/1 -> Mux2/1  "<F_zTFR>"
  Bus Selector9/3 -> Mux2/3  "<F_zTRR>"
  Bus Selector9/4 -> Mux2/4  "<F_zTRL>"
  Mux/1 -> MATLAB Function5/1(SA)
  Mux1/1 -> MATLAB Function5/2(SL)
  Mux2/1 -> MATLAB Function5/3(Fz)
  MATLAB Function5/1(F_y) -> Demux/1
  MATLAB Function5/2(F_x) -> Demux1/1
  MATLAB Function5/3(M_z) -> Demux2/1
  Demux/1 -> Bus Creator5/1  "F_yFR"
  Demux/2 -> Bus Creator5/2  "F_yFL"
  Demux/3 -> Bus Creator5/3  "F_yRR"
  Demux/4 -> Bus Creator5/4  "F_yRL"
  Demux2/2 -> Bus Creator6/2  "M_zFL"
  Demux2/3 -> Bus Creator6/3  "M_zRR"
  Demux2/4 -> Bus Creator6/4  "M_zRL"
  Demux2/1 -> Bus Creator6/1  "M_zFR"
  Demux1/4 -> Scope6/4, Bus Creator7/4  "F_xRL"
  Demux1/3 -> Scope6/3, Bus Creator7/3  "F_xRR"
  Demux1/2 -> Scope6/2, Bus Creator7/2  "F_xFL"
  Demux1/1 -> Scope6/1, Bus Creator7/1  "F_xFR"
  Bus Creator7/1 -> Bus Creator8/2  "F_x"
  Bus Creator5/1 -> Bus Creator8/1  "F_y"
  Bus Creator6/1 -> Bus Creator8/3  "M_z"
  Bus Creator8/1 -> Tyre Forces/1
  Bus Selector7/1 -> Mux/1  "<SA_FR>"
  Bus Selector7/2 -> Mux/2  "<SA_FL>"
  Bus Selector7/3 -> Mux/3  "<SA_RR>"
  Bus Selector7/4 -> Mux/4  "<SA_RL>"

== matlab function EVX_Lap_Simulation 2/EVX_Vehicle_Model/Subsystem/Chassis Vertical Initial Conditions ==
  data: Initial output
function Initial = Chassis_Vertical_Initial()
% Initial Conditions
z_c = -0.25;
y_thetaC = 0;
x_thetaCF = 0;
x_thetaCR = 0;
x_WFR = -0.04;
x_WFL = -0.04;
x_WRR = -0.04;
x_WRL = -0.04;
zdot_c = 0;
ydot_thetaC = 0;
xdot_thetaCF = 0;
xdot_thetaCR = 0;
xdot_WFR = 0;
xdot_WFL = 0;
xdot_WRR = 0;
xdot_WRL = 0;

Initial = [z_c, zdot_c,...
    y_thetaC, ydot_thetaC,...
    x_thetaCF, xdot_thetaCF,...
    x_thetaCR, xdot_thetaCR,...
    x_WFR, xdot_WFR,...
    x_WFL, xdot_WFL,...
    x_WRR, xdot_WRR,...
    x_WRL, xdot_WRL];

== matlab function EVX_Lap_Simulation 2/EVX_Vehicle_Model/Powertrain/Motor Fucntion ==
  data: Pedal input; Torque output; Motor_Speed input; Direction input
function Torque  = Motor(Pedal,Motor_Speed,Direction)

if Pedal > 100
    Pedal = 100;
elseif Pedal < 0
    Pedal = 0;
end

power = 10000;

max_torque = 50;

torque_line = abs(power / Motor_Speed) * Direction;

Torque = min(max_torque,torque_line) * (Pedal / 100);

== matlab function EVX_Lap_Simulation 2/EVX_Vehicle_Model/Powertrain/Transmission Function ==
  data: Ratio input; T_FR output; Motor_Torque input; Splits input; T_FL output; T_RR output; T_RL output
function [T_FR,T_FL,T_RR,T_RL] = Transmission(Ratio,Motor_Torque,Splits)

T_FR = 0;
T_FL = T_FR;
T_RR = (Motor_Torque * Ratio) / (Splits + 1);
T_RL = T_RR;

== matlab function EVX_Lap_Simulation 2/EVX_Vehicle_Model/Powertrain/Reverse Transmission Function ==
  data: Ratio input; Motor_Speed output; w_FR input; w_FL input; w_RR input; w_RL input
function Motor_Speed = Rev_Transmission(Ratio,w_FR,w_FL,w_RR,w_RL)

Motor_Speed = ((w_RR + w_RL) / 2) * Ratio;

== matlab function EVX_Lap_Simulation 2/EVX_Vehicle_Model/Wheel Dynamics/Wheel Acceleration Function ==
  data: F_x input; T input; I input; wdot output; r input
function wdot   = Wheel_Acceleration(F_x,T,I,r)


wdot = (T - F_x .* r)./I;

== matlab function EVX_Lap_Simulation 2/EVX_Vehicle_Model/Car_Parameters/MATLAB Function ==
  data: r_FR output; r_FL output; r_RR output; r_RL output; I_FR output; I_FL output; I_RR output; I_RL output
function [r_FR,r_FL,r_RR,r_RL,I_FR,I_FL,I_RR,I_RL] = Wheel_Parameters

r_FR = 0.175;
r_FL = 0.175;
r_RR = 0.175;
r_RL = 0.175;

I_FR = 20;
I_FL = 20;
I_RR = 20;
I_RL = 20;

== matlab function EVX_Lap_Simulation 2/EVX_Vehicle_Model/Tyre Model/Slip Ratio ==
  data: V_x input; SL output; omega_w input; r input; t input
function SL  = Slip_Ratio(V_x,omega_w,r,t)


SL = ((omega_w .* r - V_x) ./ V_x);


% if t > 1
%     pause(0.1);
% end

% if t < 0.1
%     SL(3) = 0.1;
%     SL(4) = 0.1;
%     SL(2) = 0;
%     SL(1) = 0;
% end

== matlab function EVX_Lap_Simulation 2/EVX_Vehicle_Model/Tyre Model/Slip Angle ==
  data: Vy input; Vx input; SA output; thetadot input; delta input; a input; b input; d_F input; e_F input; d_R input; e_R input
function SA  = Slip_Angle(Vy,Vx,thetadot,delta,a,b,d_F,e_F,d_R,e_R)

V_x = zeros(4);
V_y = zeros(4);
V_x = V_x(:,1);
V_y = V_y(:,1);

V_x(1) = Vx + thetadot * e_F;
V_x(2) = Vx - thetadot * d_F;
V_x(3) = Vx + thetadot * e_R;
V_x(4) = Vx - thetadot * d_R;

V_y(1) = Vy + thetadot * a;
V_y(2) = Vy + thetadot * a;
V_y(3) = Vy - thetadot * b;
V_y(4) = Vy - thetadot * b;

alpha = atand(V_y ./ V_x);

SA = delta - alpha;

== matlab function EVX_Lap_Simulation 2/EVX_Vehicle_Model/Subsystem3/Front//Rear Split ==
  data: Angle input; Steering_F output; Steering_R output
function [Steering_F,Steering_R] = Steering_Split(Angle)

Steering_F = Angle;
Steering_R = 0;

== matlab function EVX_Lap_Simulation 2/EVX_Vehicle_Model/Subsystem3/MATLAB Function ==
  data: Steering_F input; S_FR output; Ratio input; S_FL output
function [S_FR,S_FL] = Steeting_Front(Steering_F,Ratio)

S_FR = Steering_F / Ratio;
S_FL = Steering_F / Ratio;

== matlab function EVX_Lap_Simulation 2/EVX_Vehicle_Model/Subsystem3/MATLAB Function1 ==
  data: Steering_R input; S_RR output; Ratio input; S_RL output
function [S_RR,S_RL] = Steeting_Rear(Steering_R,Ratio)

S_RR = Steering_R / Ratio;
S_RL = Steering_R / Ratio;

== matlab function EVX_Lap_Simulation 2/EVX_Vehicle_Model/Tyre Model/Pacejka Tyre Model/MATLAB Function8 ==
  data: F_z input; F_xo output; SL input; SA input; gam input; F_zo input; R_wheel input; F_yo output; M_zo output; q_Bz1 input; q_Bz2 input; q_Bz3 input; q_Bz4 input; q_Bz5 input; q_Bz9 input; q_Bz10 input; q_Cz1 input; q_Dz1 input; q_Dz2 input; q_Dz3 input; q_Dz4 input; q_Dz6 input; q_Dz7 input; q_Dz8 input; q_Dz9 input; q_Ez1 input; q_Ez2 input; q_Ez3 input; q_Ez4 input; q_Ez5 input; q_Hz1 input; q_Hz2 input; q_Hz3 input; q_Hz4 input; p_Cy1 input; p_Dy1 input; p_Dy2 input; p_Dy3 input; p_Ey1 input; p_Ey2 input; p_Ey3 input; p_Ey4 input; p_Ky1 input; p_Ky2 input; p_Ky3 input; p_Hy1 input; p_Hy2 input; p_Hy3 input; p_Vy1 input; p_Vy2 input; p_Vy3 input; p_Vy4 input; p_Cx1 input; p_Dx1 input; p_Dx2 input; p_Ex1 input; p_Ex2 input; p_Ex3 input; p_Ex4 input; p_Kx1 input; p_Kx2 input; p_Kx3 input; p_Hx1 input; p_Hx2 input; p_Vx1 input; p_Vx2 input; car_mu_scaling input; run_info input
function [F_xo,F_yo,M_zo] = Pacejka_Tyre_Model(F_z,SL,SA,gam,F_zo,R_wheel,...
    q_Bz1,q_Bz2,q_Bz3,q_Bz4,q_Bz5,q_Bz9,q_Bz10,q_Cz1,q_Dz1,...
    q_Dz2,q_Dz3,q_Dz4,q_Dz6,q_Dz7,q_Dz8,q_Dz9,q_Ez1,q_Ez2,q_Ez3,q_Ez4,q_Ez5,...
    q_Hz1,q_Hz2,q_Hz3,q_Hz4,p_Cy1,p_Dy1,p_Dy2,p_Dy3,p_Ey1,p_Ey2,p_Ey3,...
    p_Ey4,p_Ky1,p_Ky2,p_Ky3,p_Hy1,p_Hy2,p_Hy3,p_Vy1,p_Vy2,p_Vy3,p_Vy4,...
    p_Cx1,p_Dx1,p_Dx2,p_Ex1,p_Ex2,p_Ex3,p_Ex4,p_Kx1,p_Kx2,p_Kx3,p_Hx1,...
    p_Hx2,p_Vx1,p_Vx2,car_mu_scaling,run_info)

dF_z = (F_z - F_zo) ./ (F_zo);

lamda_mux = 1;

%% Longitudinal Force (pure longitudinal slip)
S_Vx = F_z .* (p_Vx1 + p_Vx2 .* dF_z);
S_Hx = (p_Hx1 + p_Hx2 .* dF_z);
K_xk = F_z .* (p_Kx1 + p_Kx2 .* dF_z) .* exp(p_Kx3 .* dF_z);
mu_x = (p_Dx1 + p_Dx2 .* dF_z) .* lamda_mux;
%mu_x = (sign(mu_x) + 1) / 2;
D_x = mu_x .* F_z;
%D_x = (sign(D_x) + 1) / 2;
C_x = p_Cx1;
%C_x = (sign(C_x) + 1) / 2;
B_x = K_xk ./ (C_x .* D_x);
kappa_x = SL + S_Hx;
E_x = (p_Ex1 + p_Ex2 .* dF_z + p_Ex3 .* dF_z .^2) .* (1 - p_Ex4 .* sign(kappa_x));
F_xo = D_x .* sin(C_x .* atan(B_x .* kappa_x - E_x .* (B_x .* kappa_x - atan(B_x .* kappa_x)))) + S_Vx;
    
%% Lateral Force (pure side slip)
S_Vy = F_z .* ((p_Vy1 + p_Vy2 .* dF_z) + (p_Vy3 + p_Vy4 .* dF_z) .* gam);
S_Hy = (p_Hy1 + p_Hy2 .* dF_z) + p_Hy3 .* gam;
K_yalphao = p_ky1 .* F_zo .* sin(2 .* atan(F_z ./ (p_Ky2 .* F_zo)));
K_yalpha = K_yalphao .* (1 - p_Ky3 .* gam .^2);
mu_y = (p_Dy1 + p_Dy2 .* dF_z) .* (1 - p_Dy3 .* gam .^2) .* lamda_muy;
D_y = mu_y .* F_z;
C_y = p_Cy1;
B_y = K_yalpha ./ (C_y * D_y);
alpha_y = SA + S_Hy;
E_y = (p_Ey1 + p_Ey2 .* dF_z) .* (1 - (p_Ey3 + pEy2 .* gam) .* sign(alpha_y));
F_yo = D_y .* sin(C_y .* atan(B_y .* aplha_y - E_y .* (B_y .* alpha_y - atan(B_y .* alpha_y)))) + S_Vy;

%% Longitudinal Force (Combined Slip)
% needs more coefficients

%% Lateral Force (Combined Slip)
% needs more coefficients

%% Aligning Torque (pure side slip)
S_Hf = S_Hy + S_Vy ./ K_yalpha;
alpha_r = SA + S_Hf;
B_r = q_Bz10 .* B_y .* C_y;
C_r = 1;
D_r = F_z .* R_wheel .* ((q_Dz6 + q_Dz7 .* dF_z) + (q_Dz8 + q_Dz9 .* dF_z) .* gam) .* lamda_muy;
M_zro = D_r .* cos(C_r .* atan(B_r .* alpha_r));
S_Ht = q_Hz1 + q_Hz2 .* dF_z + (q_Hz3 + q_Hz4 .* dF_z) .* gam;
alpha_t = SA + S_Ht;
B_t = (q_Bz1 + q_Bz2 .* dF_z + q_Bz2 .* dF_z .^2) .* (1 + q_Bz4 .* gam + q_Bz2 .* abs(gam)) ./ lamda_muy;
C_t = q_Cz1;
D_to = F_z .* (R_wheel ./ F_zo) .* (q_Dz1 + q_Dz2 .* dF_z);
D_t = D_to .* (1 + q_Dz3 .* gam + q_Dz3 .* gam .^2);
E_t = (q_Ez1 + q_Ez2 .* dF_z + q_Ez3 .* DF_z .^2) .* (1 + (q_Ez4 + q_Ez5 .* gam) .* (2/pi) .* atan(B_t .* C_t .* alpha_t));
t_o = D_t .* cos(C_t .* atan(B_t .* alpha_t - E_t .* (B_t .* alpha_t - atan(B_t .* alpha_t))));
Mdash_zo = -t_o .* F_yo;
M_zo = Mdash_zo + M_zro;


end

== matlab function EVX_Lap_Simulation 2/EVX_Vehicle_Model/Tyre Model/MATLAB Function ==
  data: V_y input; V_x input; V_xFR output; omega input; a input; b input; d_F input; e_F input; d_R input; e_R input; V_xFL output; V_xRR output; V_xRL output; V_yFR output; V_yFL output; V_yRR output; V_yRL output
function [V_xFR,V_xFL,V_xRR,V_xRL,V_yFR,V_yFL,V_yRR,V_yRL]...
    = Wheel_Velocities(V_y,V_x,omega,a,b,d_F,e_F,d_R,e_R)

% Wheel velocities in x direction
V_xFR = V_x + omega * e_F;
V_xFL = V_x - omega * d_F;
V_xRR = V_x + omega * e_R;
V_xRL = V_x - omega * d_R;

% Wheel velocities in y direction
V_yFR = V_y + omega * a;
V_yFL = V_y + omega * a;
V_yRR = V_y - omega * b;
V_yRL = V_y - omega * b;

== matlab function EVX_Lap_Simulation 2/EVX_Vehicle_Model/Tyre Model/Pacejka Tyre Model/MATLAB Function ==
  data: F_z input; F_yo output; mu_scaling input; SA input; SL input; F_xo output; M_zo output
function [F_yo,F_xo,M_zo] = Basic_Tyre(F_z,mu_scaling,SA,SL)

F_xo = F_z .* mu_scaling .* SL;
F_yo = F_z .* mu_scaling .* SA;
M_zo = F_z .* mu_scaling .* SA ./ 100;

== matlab function EVX_Lap_Simulation 2/EVX_Vehicle_Model/Tyre Model/Pacejka Tyre Model/MATLAB Function1 ==
  data: F_z input; F_yo output; mu_scaling input; SA input; SL input; F_xo output; M_zo output
function [F_yo,F_xo,M_zo] = Basic_Tyre(F_z,mu_scaling,SA,SL)

F_xo = F_z * mu_scaling * SL;
F_yo = F_z * mu_scaling * SA;
M_zo = F_z * mu_scaling * SA / 100;

== matlab function EVX_Lap_Simulation 2/EVX_Vehicle_Model/Tyre Model/Pacejka Tyre Model/MATLAB Function2 ==
  data: F_z input; F_yo output; mu_scaling input; SA input; SL input; F_xo output; M_zo output
function [F_yo,F_xo,M_zo] = Basic_Tyre(F_z,mu_scaling,SA,SL)

F_xo = F_z * mu_scaling * SL;
F_yo = F_z * mu_scaling * SA;
M_zo = F_z * mu_scaling * SA / 100;

== matlab function EVX_Lap_Simulation 2/EVX_Vehicle_Model/Tyre Model/Pacejka Tyre Model/MATLAB Function3 ==
  data: F_z input; F_yo output; mu_scaling input; SA input; SL input; F_xo output; M_zo output
function [F_yo,F_xo,M_zo] = Basic_Tyre(F_z,mu_scaling,SA,SL)

F_xo = F_z * mu_scaling * SL;
F_yo = F_z * mu_scaling * SA;
M_zo = F_z * mu_scaling * SA / 100;

== matlab function EVX_Lap_Simulation 2/EVX_Vehicle_Model/Car_Parameters/MATLAB Function17 ==
  data: m_C output; m_CF output; m_CR output; m_WFR output; m_WFL output; m_WRR output; m_WRL output; I_Cy output; I_CFx output; I_CRx output; I_z output; a output; b output; d_F output; e_F output; d_R output; e_R output; k_C output; c_C output; h_C output; h_CF output; h_CR output; mu_scaling output
function [m_C,m_CF,m_CR,m_WFR,m_WFL,m_WRR,m_WRL,I_Cy,I_CFx,I_CRx,I_z,a,b,d_F,...
    e_F,d_R,e_R,k_C,c_C,h_C,h_CF,h_CR,mu_scaling] = Car_Parameters
%% Car Parameters
% Masses
m_C = 250; %car sprung mass (kg)
m_CF = 100;
m_CR = m_C - m_CF;
m_WFR = 5; %front right wheel mass (kg)
m_WFL = 5; %front left wheel mass (kg)
m_WRR = 5; %rear right wheel mass (kg)
m_WRL = 5; %rear left wheel mass (kg)

% Intertias
I_Cy = 1000; %chassis interia around y (kg m^2)
I_CFx = 500; %chassis front inertia around x (kg m^2)
I_CRx = 500; %chassis rear inertia around x (kg m^2)
I_z = 2000;

% Geometries
a = 0.8; %distance of COG from front axle (m)
b = 0.8; %distance of COG from rear axle (m)
d_F = 0.6; %distance of COG from front left tire (m)
e_F = 0.6; %distance of COG from front right tire (m)
d_R = 0.6; %distance of COG from rear left tire (m)
e_R = 0.6; %distance of COG from rear right tire (m)
h_C = 0.3;
h_CF = 0.3;
h_CR = 0.3;

% Other Stiffnesses
k_C = 2000;

% Other Damping Coefficients
c_C = 1000;

% mu
mu_scaling = 0.55;

== matlab function EVX_Lap_Simulation 2/EVX_Vehicle_Model/Tyre Model/Pacejka Tyre Model/MATLAB Function4 ==
  data: F_z input; F_yo output; mu_scaling input; SA input; SL input; F_xo output; M_zo output
function [F_yo,F_xo,M_zo] = Basic_Tyre(F_z,mu_scaling,SA,SL)

F_xo = F_z * mu_scaling * SL;
F_yo = F_z * mu_scaling * SA;
M_zo = F_z * mu_scaling * SA / 100;

== matlab function EVX_Lap_Simulation 2/EVX_Vehicle_Model/Tyre Model/Slip Ratio1 ==
  data: V_xFR input; SL_FR output; V_xFL input; SL_FL output; SL_RR output; SL_RL output; V_xRR input; V_xRL input; omega_wFR input; omega_wFL input; omega_wRR input; omega_wRL input; r_FR input; r_FL input; r_RR input; r_RL input; t input
function [SL_FR,SL_FL,SL_RR,SL_RL] = Slip_Ratio(V_xFR,V_xFL,V_xRR,V_xRL,...
    omega_wFR,omega_wFL,omega_wRR,omega_wRL,r_FR,r_FL,r_RR,r_RL,t)

if V_xFR == 0
    if omega_wFR > 0
        SL_FR = 1;
    elseif omega_wFR < 0
        SL_FR = -1;
    else
        SL_FR = 0;
    end
else
    SL_FR = ((omega_wFR * r_FR) / V_xFR) - 1;
end
    
if V_xFL == 0
    if omega_wFL > 0
        SL_FL = 1;
    elseif omega_wFL < 0
        SL_FL = -1;
    else
        SL_FL = 0;  
    end
else
    SL_FL = ((omega_wFL * r_FL) / V_xFL) - 1;
end

if V_xRR == 0
    if omega_wRR > 0
        SL_RR = 1;
    elseif omega_wRR < 0
        SL_RR = -1;
    else
        SL_RR = 0;  
    end
else
    SL_RR = ((omega_wRR * r_RR) / V_xRR) - 1;
end

if V_xRL == 0
    if omega_wRL > 0
        SL_RL = 1;
    elseif omega_wRL < 0
        SL_RL = -1;
    else
        SL_RL = 0;  
    end
else
    SL_RL = ((omega_wRL * r_RL) / V_xRL) - 1;
end

if SL_FR > 1
    SL_FR = 1;
end

if SL_FL > 1
    SL_FL = 1;
end

if SL_RR > 1
    SL_RR = 1;
end

if SL_RL > 1
    SL_RL = 1;
end

if SL_FR < -1
    SL_FR = -1;
end

if SL_FL < -1
    SL_FL = -1;
end

if SL_RR < -1
    SL_RR = -1;
end

if SL_RL < -1
    SL_RL = -1;
end

% if t > 1
%     pause(0.1);
% end

if t < 0.1
    SL_RR = 1;
    SL_RL = 1;
    SL_FR = 0;
    SL_FL = 0;
end

== matlab function EVX_Lap_Simulation 2/EVX_Vehicle_Model/Chassis Vertical Dynamics/MATLAB Function19 ==
  data: Z output; z input; m_C input; m_WFR input; m_WFL input; m_WRR input; m_WRL input; I_Cy input; I_CFx input; I_CRx input; a input; b input; d_F input; e_F input; d_R input; e_R input; k_C input; c_C input; k_SFR input; k_SFL input; k_SRR input; k_SRL input; k_TFR input; k_TFL input; k_TRR input; k_TRL input; c_SFR input; c_SFL input; c_SRR input; c_SRL input; c_TFR input; c_TFL input; c_TRR input; c_TRL input; F_zC input; M_y input; M_xF input; M_xR input; F_zWFR input; F_zWFL input; F_zWRR input; F_zWRL input; y_FR input; y_FL input; y_RR input; y_RL input; ydot_FR input; ydot_FL input; ydot_RR input; ydot_RL input
function Z = Chassis8(z,m_C,m_WFR,m_WFL,m_WRR,m_WRL,...
    I_Cy,I_CFx,I_CRx,a,b,d_F,e_F,d_R,e_R,k_C,c_C,k_SFR,k_SFL,k_SRR,k_SRL,...
    k_TFR,k_TFL,k_TRR,k_TRL,c_SFR,c_SFL,c_SRR,c_SRL,c_TFR,c_TFL,...
    c_TRR,c_TRL,F_zC,M_y,M_xF,M_xR,F_zWFR,F_zWFL,F_zWRR,F_zWRL,y_FR,...
    y_FL,y_RR,y_RL,ydot_FR,ydot_FL,ydot_RR,ydot_RL)

Z = [z(2);...
    ...
    (1/m_C) * (F_zC...
    + k_SRR * (z(9) - z(1) - b * z(3) + e_R * z(7))...
    + k_SFR * (z(11) - z(1) + a * z(3) + e_F * z(5))...
    + k_SFL * (z(13) - z(1) + a * z(3) - d_F * z(5))...
    + k_SRL * (z(15) - z(1) - b * z(3) - d_R * z(7))...
    + c_SRR * (z(10) - z(2) - b * z(4) + e_R * z(8))...
    + c_SFR * (z(12) - z(2) + a * z(4) + e_F * z(6))...
    + c_SFL * (z(14) - z(2) + a * z(4) - d_F * z(6))...
    + c_SRL * (z(16) - z(2) - b * z(4) - d_R * z(8)));...
    ...
    z(4);...
    ...
    (1/I_Cy) * (M_y...
    + b * k_SRR * (z(9) - z(1) - b * z(3) + e_R * z(7))...
    - a * k_SFR * (z(11) - z(1) + a * z(3) + e_F * z(5))...
    - a * k_SFL * (z(13) - z(1) + a * z(3) - d_F * z(5))...
    + b * k_SRL * (z(15) - z(1) - b * z(3) - d_R * z(7))...
    + b * c_SRR * (z(10) - z(2) - b * z(4) + e_R * z(8))...
    - a * c_SFR * (z(12) - z(2) + a * z(4) + e_F * z(6))...
    - a * c_SFL * (z(14) - z(2) + a * z(4) - d_F * z(6))...
    + b * c_SRL * (z(16) - z(2) - b * z(4) - d_R * z(8)));...
    ...
    z(6);...
    ...
    (1/I_CFx) * (M_xF...
    - e_F * k_SFR * (z(11) - z(1) + a * z(3) + e_F * z(5))...
    + d_F * k_SFL * (z(13) - z(1) + a * z(3) - d_F * z(5))...
    - k_C * (z(5) - z(7))...
    - e_F * c_SFR * (z(12) - z(2) + a * z(4) + e_F * z(6))...
    + d_F * c_SFL * (z(14) - z(2) + a * z(4) - d_F * z(6))...
    - c_C * (z(6) - z(8)));...
    ...
    z(8);...
    ...
    (1/I_CRx) * (M_xR...
    - e_R * k_SRR * (z(9) - z(1) - b * z(3) + e_R * z(7))...
    + d_F * k_SRL * (z(15) - z(1) - b * z(3) - d_R * z(7))...
    + k_C * (z(5) - z(7))...
    - e_R * c_SRR * (z(10) - z(2) - b * z(4) + e_R * z(8))...
    + d_F * c_SRL * (z(16) - z(2) - b * z(4) - d_R * z(8))...
    + c_C * (z(6) - z(8)));...
    ...
    z(10);...
    ...
    (1/m_WRR) * (F_zWRR...
    + k_TRR * (y_RR - z(9))...
    - k_SRR * (z(9) - z(1) - b * z(3) + e_R * z(7))...
    + c_TRR * (ydot_RR - z(10))...
    - c_SRR * (z(10) - z(2) - b * z(4) + e_R * z(8)));...
    ...
    z(12);...
    ...
    (1/m_WFR) * (F_zWFR...
    + k_TFR * (y_FR - z(11))...
    - k_SFR * (z(11) - z(1) + a * z(3) + e_F * z(5))...
    + c_TFR * (ydot_FR - z(12))...
    - c_SFR * (z(12) - z(2) + a * z(4) + e_F * z(6)));...
    ...
    z(14);...
    ...
    (1/m_WFL) * (F_zWFL...
    + k_TFL * (y_FL - z(13))...
    - k_SFL * (z(13) - z(1) + a * z(3) - d_F * z(5))...
    + c_TFL * (ydot_FL - z(14))...
    - c_SFL * (z(14) - z(2) + a * z(4) - d_F * z(6)));...
    ...
    z(16);...
    ...
    (1/m_WRL) * (F_zWRL...
    + k_TRL * (y_RL - z(15))...
    - k_SRL * (z(15) - z(1) - b * z(3) - d_R * z(7))...
    + c_TRL * (ydot_RL - z(16))...
    - c_SRL * (z(16) - z(2) - b * z(4) - d_R * z(8)))...
    ];

end

== matlab function EVX_Lap_Simulation 2/EVX_Vehicle_Model/Horizontal Dynamics/MATLAB Function18 ==
  data: g input; a_y output; m_C input; h_C input; m_CF input; m_CR input; h_CF input; h_CR input; a input; b input; d_F input; e_F input; d_R input; e_R input; F_yFR input; F_yFL input; F_yRR input; F_yRL input; F_xFR input; F_xFL input; F_xRR input; F_xRL input; M_zFR input; M_zFL input; M_zRR input; M_zRL input; S_FR input; S_FL input; S_RR input; S_RL input; m_WRL input; m_WRR input; m_WFL input; m_WFR input; a_x output; thetaddot_z output; M_y output; M_xF output; M_xR output; F_z output; I_z input; F_Ad input; F_Az input
function [a_y,a_x,thetaddot_z,M_y,M_xF,M_xR,F_z] = Chassis7(g,m_C,h_C,m_CF,m_CR,...
    h_CF,h_CR,a,b,d_F,e_F,d_R,e_R,F_yFR,F_yFL,F_yRR,F_yRL,F_xFR,F_xFL,...
    F_xRR,F_xRL,M_zFR,M_zFL,M_zRR,M_zRL,S_FR,S_FL,S_RR,S_RL,m_WRL,m_WRR,...
    m_WFL,m_WFR,I_z,F_Ad,F_Az)

F_y = F_yRL * cos(S_RL) + F_yRR * cos(S_RR) + F_yFL * cos(S_FL) + ...
    F_yFR * cos(S_FR)...
     - F_xRL * sin(S_RL) - F_xRR * sin(S_RR) + F_xFL * sin(S_FL) + ...
    F_xFR * sin(S_FR);

F_x = -F_Ad + F_xRL * cos(S_RL) + F_xRR * cos(S_RR) + F_xFL * cos(S_FL) + ...
    F_xFR * cos(S_FR)...
     + F_yRL * sin(S_RL) + F_yRR * sin(S_RR) - F_yFL * sin(S_FL) - ...
    F_yFR * sin(S_FR);

F_z = -F_Az - g * m_C;

M_z = F_xRR * (sin(S_RR) * b + cos(S_RR) * e_R) +...
    F_yRR * (sin(S_RR) * e_R - cos(S_RR) * b) +...
    F_xFR * (cos(S_FR) * e_F + sin(S_FR) * a) +...
    F_yFR * (cos(S_FR) * a - sin(S_FR) * e_F) +...
    F_xFL * (-cos(S_FL) * d_F + sin(S_FL) * a) +...
    F_yFL * (cos(S_FL) * a + sin(S_FL) * d_F) +...
    F_xRL * (-cos(S_RL) * d_R + sin(S_RL) * b) +...
    F_yRL * (-sin(S_RL) * d_R - cos(S_RL) * b) +...
    + M_zFL + M_zRL + M_zRR + M_zFR;

m = m_C + m_WRL + m_WRR + m_WFL + m_WFR;
a_x = F_x / m;
a_y = F_y / m;
thetaddot_z = M_z / I_z;
M_y = -m_C * a_x * h_C;
M_xF = m_CF * a_y * h_CF;
M_xR = m_CR * a_y * h_CR;
